simulink library "library_ALICAT_BASIS_RW"  (R2024b)
settings: Solver=VariableStepAuto  StartTime=0.0  StopTime=10.0  RelTol=1e-3
undefined symbols (not defined in the file): Controller
settings Model: Creator=GavinWilliamson  LastModifiedBy=GavinWilliamson

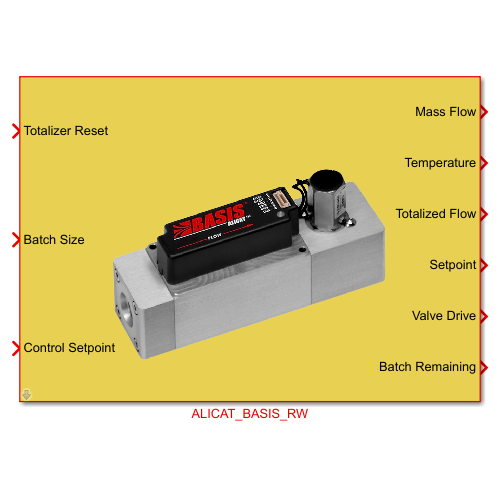
[thumbnail: Simulink's stored preview of the top-level diagram]
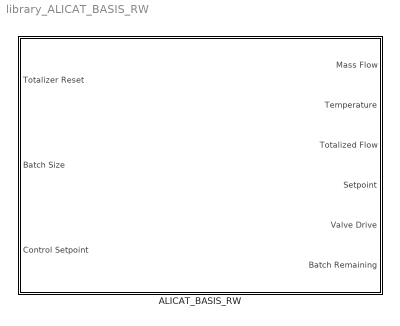
== system library_ALICAT_BASIS_RW ==
  ALICAT_BASIS_RW : Subsystem  mask{Port="COM5", Device_Name='A', gs_type=Hydrogen, dv_typ=Controller, contrl_typ=Mass Flow, batch_sw=on}
      mask prompts: Device_Name "Device Identifier"; gs_type "Gas Type"; dv_typ "Device Type"; contrl_typ "Setpoint Variable"; batch_sw "Enable Batching"
      mask help: Default Mask
      mask Help: web(which('help_ALICAT_BASIS_RW.html'), '-helpbrowser')
      mask TypeOptions Port:
      | Level-2 MATLAB
      | S-Function/Port
      mask TypeOptions Device_Name:
      | Level-2 MATLAB
      | S-Function/Device_Name
      mask TypeOptions gs_type:
      | Level-2 MATLAB
      | S-Function/gs_type
      mask TypeOptions dv_typ:
      | Level-2 MATLAB
      | S-Function/dv_typ
      mask TypeOptions contrl_typ:
      | Level-2 MATLAB
      | S-Function/contrl_typ
      mask TypeOptions batch_sw:
      | Level-2 MATLAB
      | S-Function/batch_sw
      mask DialogControl Container3 Prompt: General
      mask DialogControl Container5 Prompt: ALICAT_BASIS_RW
      mask DialogControl Control1 Prompt: Block controls and reads an ALICAT BASIS devices over serial communication. Labels on the ports on the block will disappear if there are not valid for the configuration selected. To see all port labels you can look under the mask of this block.
      mask DialogControl Container6 Prompt: Communciation Parameters
      mask DialogControl Container7 Prompt: Control Options
      mask DialogControl Container4 Prompt: Instructions
      mask DialogControl Container8 Prompt: Inputs
      mask DialogControl Control2 Prompt: Totalizer Reset: Input should be a constant block that is set to 0. A push button should be linked to the block to change the value to 1 when pushed. When the button is pushed the totalizer will then be reset.
      mask DialogControl Control3 Prompt: Batch Limit: The input for totalizer limit will only be written to the device if the totalizer and batching are enabled in the register parameters.
      mask DialogControl Container9 Prompt: Register Parameters
      mask DialogControl Container10 Prompt: Communication Parameters
      mask DialogControl Control4 Prompt: Port: Communication port that ALICAT is connected to [string]
      mask DialogControl Control5 Prompt: Device Identifier: Unit ID of ALICAT [char]
      mask DialogControl Container11 Prompt: Gas Type
      mask DialogControl Control7 Prompt: Process gas flowing through ALICAT
      mask DialogControl Container12 Prompt: Device Type
      mask DialogControl Control8 Prompt: Select whether the ALICAT that is connected to the COM Port is a controller or meter. This is important to ensure invalid commands are not sent to the device, and to ensure that the outputted data is in the expected format.
      mask DialogControl Container13 Prompt: Control Options
      mask DialogControl Control9 Prompt: Setpoint Variable: If set to "Valve Drive", "Control Setpoint" should be set to the percentage open on the range of 0-100. Where 0 corresponds to closed and 100 corresponds to fully open.
      mask DialogControl Control10 Prompt: Enable Batching: This enables the batching on the ALICAT and enables the batch limit to be updated while the model is running.
      mask Display:
      | image('BASIS-controller-prod-600px.png', [20,20,20,20,100,100]);
      | 
      | %input ports
      | port_label('input', 1, 'Totalizer Reset');
      | if strcmp(get_param(gcb,'batch_sw'),'on')
      |     port_label('input', 2, 'Batch Size');
      | end
      | if strcmp(get_param(gcb,'dv_typ'),'Controller')
      |     port_label('input', 3, 'Control Setpoint');
      | end
      | 
      | %output ports
      | port_label('output', 1, 'Mass Flow');
      | port_label('output', 2, 'Temperature');
      | port_label('output', 3, 'Totalized Flow');
      | if strcmp(get_param(gcb,'dv_typ'),'Controller')
      |     port_label('output', 4, 'Setpoint');
      |     port_label('output', 5, 'Valve Drive');
      | end
      | if strcmp(get_param(gcb,'batch_sw'),'on')
      |     port_label('output', 6, 'Batch Remaining');
      | end

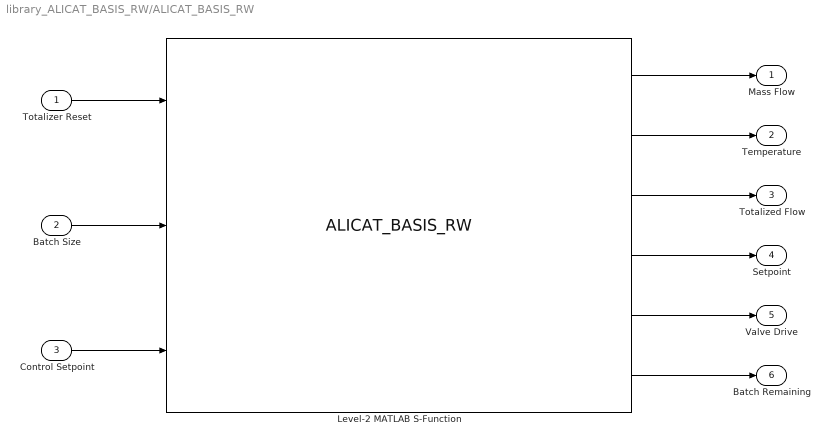
== system library_ALICAT_BASIS_RW/ALICAT_BASIS_RW ==
  Totalizer Reset : Inport
  Batch Size : Inport  Port=2
  Control Setpoint : Inport  Port=3
  Level-2 MATLAB S-Function : M-S-Function  FunctionName=ALICAT_BASIS_RW  Parameters=Port, Device_Name, gs_type, batch_sw, contrl_typ, dv_typ  mask{Port=Port, Device_Name=Device_Name, gs_type=Hydrogen, dv_typ=Controller, contrl_typ=Mass Flow, batch_sw=on}
      mask prompts: Device_Name "Device Identifier"; gs_type "Gas Type"; dv_typ "Device Type"; contrl_typ "Setpoint Variable"; batch_sw "Enable Batching"
      mask TypeOptions gs_type: Hydrogen | Nitrogen | Air
      mask TypeOptions dv_typ: Controller | Meter
      mask TypeOptions contrl_typ: Mass Flow | Valve Drive
      mask DialogControl DescGroupVar Prompt: ALICAT__BASIS_RW
      mask DialogControl DescTextVar Prompt: *See mask of subsystem
      mask DialogControl Container4 Prompt: Connection Parameters
      mask DialogControl Container6 Prompt: Control Options
      mask Display:
      | image('BASIS-controller-prod-600px.png', [20,20,20,20,100,100]);
      | 
      | 
      | port_label('input', 1, 'Totalizer Reset');
      | port_label('input', 2, 'Batch Size');
      | port_label('input', 3, 'Control Setpoint');
      | 
      | port_label('output', 1, 'Mass Flow');
      | port_label('output', 2, 'Temperature');
      | port_label('output', 3, 'Totalized Flow');
      | port_label('output', 4, 'Setpoint');
      | port_label('output', 5, 'Valve Drive');
      | port_label('output', 6, 'Batch Remaining');
  Mass Flow : Outport
  Temperature : Outport  Port=2
  Totalized Flow : Outport  Port=3
  Setpoint : Outport  Port=4
  Valve Drive : Outport  Port=5
  Batch Remaining : Outport  Port=6
  wires:
  Totalizer Reset/1 -> Level-2 MATLAB S-Function/1
  Batch Size/1 -> Level-2 MATLAB S-Function/2
  Control Setpoint/1 -> Level-2 MATLAB S-Function/3
  Level-2 MATLAB S-Function/1 -> Mass Flow/1
  Level-2 MATLAB S-Function/3 -> Totalized Flow/1
  Level-2 MATLAB S-Function/2 -> Temperature/1
  Level-2 MATLAB S-Function/4 -> Setpoint/1
  Level-2 MATLAB S-Function/5 -> Valve Drive/1
  Level-2 MATLAB S-Function/6 -> Batch Remaining/1
